simulink model "slider_mode_controller"  (R2021b)
settings: Solver=VariableStepAuto  StartTime=0.0  StopTime=1000  RelTol=1e-3
settings Model: Creator=alefr  LastModifiedBy=alefr

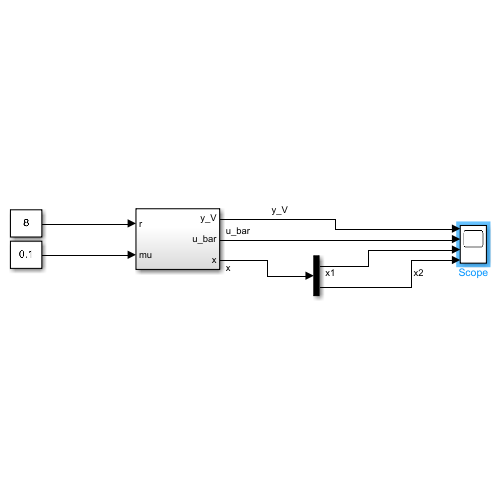
[thumbnail: Simulink's stored preview of the top-level diagram]
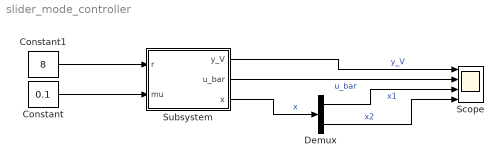
== system slider_mode_controller ==
  Constant : Constant  Value=0.1
  Constant1 : Constant  Value=8
  Demux : Demux  Outputs=2
  Scope : Scope  NumInputPorts=4
  Subsystem : Subsystem
  wires:
  Subsystem/1(y_V) -> Scope/1  "y_V"
  Subsystem/3(x) -> Demux/1  "x"
  Demux/2 -> Scope/4  "x2"
  Subsystem/2(u_bar) -> Scope/2  "u_bar"
  Demux/1 -> Scope/3  "x1"
  Constant/1 -> Subsystem/2(mu)
  Constant1/1 -> Subsystem/1(r)

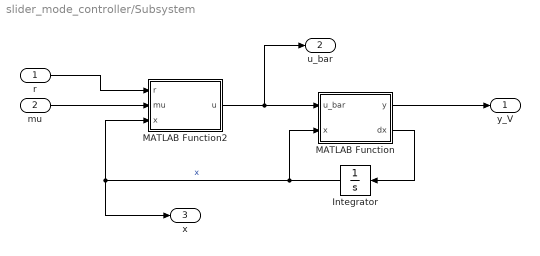
== system slider_mode_controller/Subsystem ==
  r : Inport
  mu : Inport  Port=2
  Integrator : Integrator  InitialCondition=[8;8]
  MATLAB Function : MATLAB Function  TreatAsAtomicUnit=on
  MATLAB Function2 : MATLAB Function  TreatAsAtomicUnit=on
  y_V : Outport
  u_bar : Outport  Port=2
  x : Outport  Port=3
  wires:
  Integrator/1 -> MATLAB Function/2(x), MATLAB Function2/3(x), x/1  "x"
  MATLAB Function/1(y) -> y_V/1
  MATLAB Function/2(dx) -> Integrator/1
  MATLAB Function2/1(u) -> MATLAB Function/1(u_bar), u_bar/1
  mu/1 -> MATLAB Function2/2(mu)
  r/1 -> MATLAB Function2/1(r)

== matlab function slider_mode_controller/Subsystem/MATLAB Function2 ==
  data: r input; mu input; u output; x input
function u = fcn(r,mu,x)

x1=x(1);
x2=x(2);
u = sqrt(2.0).*sqrt(x1.*5.0+1.6e+1).*((sqrt(2.0).*(sqrt(x1.*5.0+1.6e+1).*7.609042393596842e-2-sqrt(x2.*5.0+1.6e+1).*7.609042393596842e-2))./2.0+sqrt(2.0).*1.0./sqrt(x1.*5.0+1.6e+1).*1.0./sqrt(x2.*5.0+1.6e+1).*(x1.*2.7795e+4+8.8944e+4).*1.74599430814118e-6).*(-1.734778086018821e+2)-sqrt(2.0).*mu.*sqrt(x1.*5.0+1.6e+1).*min([1.0,max([-1.0,-r+x2.*7.456422751238219e-1+sqrt(x1.*1.962e+3+6.2784e+3).*3.841187477910597e-3-sqrt(x2.*1.962e+3+6.2784e+3).*3.841187477910597e-3-1.648066384406454],[],2,'omitnan')],[],2,'omitnan').*1.734778086018821e+2;
end

== matlab function slider_mode_controller/Subsystem/MATLAB Function ==
  data: u_bar input; y output; x input; dx output
function [y,dx] = fcn(u_bar,x)

x1 = x(1);
x2 = x(2);

dx = [u_bar./3.3e+1-sqrt(x1.*1.962e+3+6.2784e+3).*5.151515151515152e-3;
    sqrt(x1.*1.962e+3+6.2784e+3).*5.151515151515152e-3-sqrt(x2.*1.962e+3+6.2784e+3).*5.151515151515152e-3];

y = x2.*7.456422751238219e-1-1.648066384406454;

end
